simulink model "DPT"  (R2025b)
settings: Solver=VariableStepAuto  StartTime=0.0  StopTime=10  RelTol=1e-3
undefined symbols (not defined in the file): J, k_M, k_n, L_a, R_a
libraries: simulink x1
settings Model: Creator=user  LastModifiedBy=user

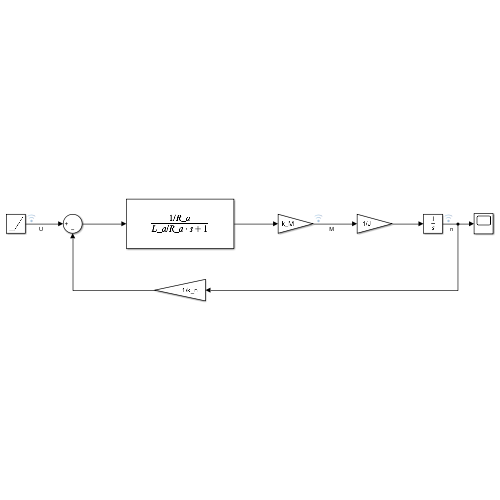
[thumbnail: Simulink's stored preview of the top-level diagram]
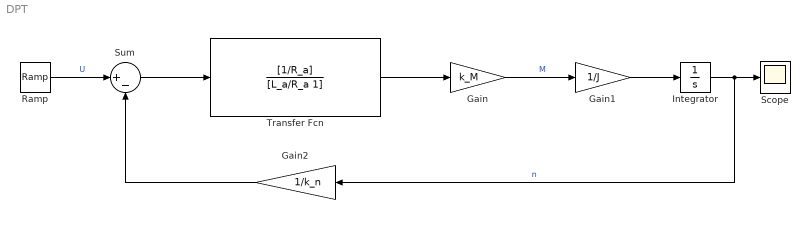
== system DPT ==
  Gain : Gain  Gain=k_M
  Gain1 : Gain  Gain=1/J
  Gain2 : Gain  Gain=1/k_n
  Integrator : Integrator
  Ramp : simulink/Sources/Ramp  slope=2.4  start=0  InitialOutput=0
  Scope : Scope
      settings: ActiveDisplayYMinimum=-1103.7717534389949  ActiveDisplayYMaximum=9933.9457809509568
  Sum : Sum  Inputs=|+-
  Transfer Fcn : TransferFcn  Numerator=[1/R_a]  Denominator=[L_a/R_a 1]
  wires:
  Sum/1 -> Transfer Fcn/1
  Transfer Fcn/1 -> Gain/1
  Gain/1 -> Gain1/1  "M"
  Gain1/1 -> Integrator/1
  Gain2/1 -> Sum/2
  Integrator/1 -> Gain2/1, Scope/1  "n"
  Ramp/1 -> Sum/1  "U"
